simulink model "ShortPulse"  (R2018a)
settings: Solver=ode8  StartTime=0.0  StopTime=Ttot  FixedStep=Ts  RelTol=1e-3
values from neighbouring files (symbols this model uses):
  Fn = 60    [Equivalency_Script.m]    (also in FreqAdaptiveFFT_Script.m; FreqAdaptive_Script.m; ShortPulse_Script.m)
  Ts = Ts_control / 60    (= 9.25925925926e-07)    [Equivalency_Script.m]    (also in FreqAdaptiveFFT_Script.m; FreqAdaptive_Script.m; ShortPulse_Script.m)
  Ts_control = 1/(300*Fn)    (= 5.55555555556e-05)    [Equivalency_Script.m]    (also in FreqAdaptiveFFT_Script.m; FreqAdaptive_Script.m; ShortPulse_Script.m)
libraries: powerlib x3, DSCdq_Library x3, powerlib_meascontrol x1
settings Model: SimulationMode=accelerator  Creator=daniemot  LastModifiedBy=daniemot
settings SolverCC: AutoInsertRateTranBlk=on
settings DataIOCC: ExternalInput=getinputstruct(WN_50mF_op_snapshot1)  InitialState=getstatestruct(WN_50mF_op_snapshot1)  SaveFinalState=on  SaveFormat=StructureWithTime  SaveOutput=off  SignalLogging=off  DSMLogging=off  SaveTime=off
settings DebuggingCC: ReadBeforeWriteMsg=DisableAll  WriteAfterWriteMsg=DisableAll  WriteAfterReadMsg=DisableAll  MultiTaskDSMMsg=none  UnconnectedInputMsg=none  UnconnectedOutputMsg=none  UnconnectedLineMsg=none
settings ModelReferenceCC: UpdateModelReferenceTargets=IfOutOfDate
settings SFSimCC: SFSimEcho=off

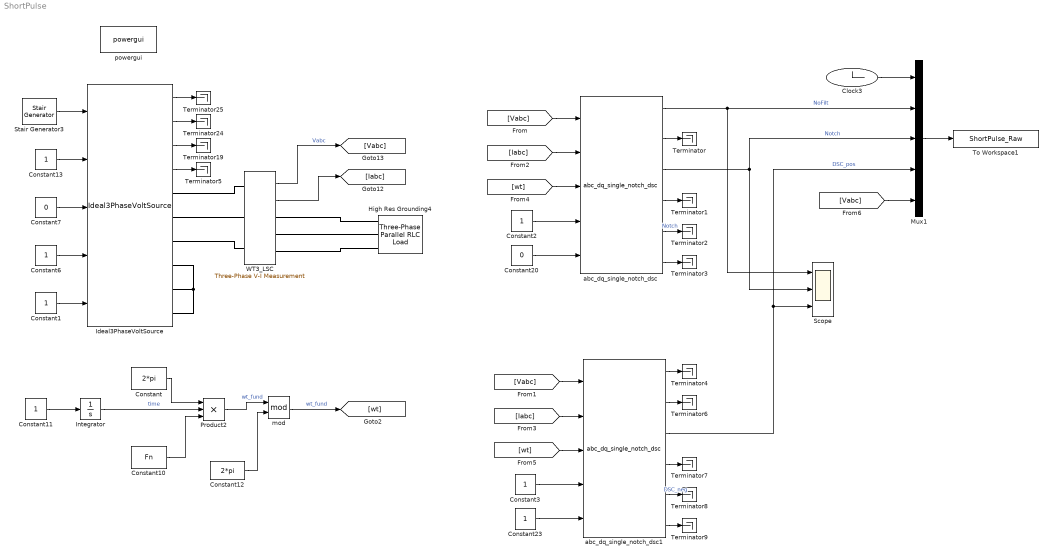
== system ShortPulse ==
  Clock3 : Clock
  Constant : Constant  Value=2*pi
  Constant{1..3,6,11,13,23} (7 alike) : Constant
  Constant10 : Constant  Value=Fn
  Constant12 : Constant  Value=2*pi
  Constant20 : Constant  Value=0
  Constant7 : Constant  Value=0
  High Res Grounding4 : powerlib/Elements/Three-Phase Parallel RLC Load  LConnTagsString=A|B|C  Configuration=Y (grounded)  NominalVoltage=(1/2^0.5)*3^0.5  Vabc=[1e3 1e3 1e3]  Vabcp=[1e3 1e3 1e3]  NominalFrequency=Fn  UnbalancedPower=off  ActivePower=3/2  InductivePower=0  CapacitivePower=0  Pabc=[10e3 9e3 11e3]  QLabc=[100 90 110]  QCabc=[100 90 110]  Pabcp=[10e3 9e3 11e3]  QLabcp=[100 90 110]  QCabcp=[100 90 110]  Measurements=None  LoadType=constant Z
  Ideal3PhaseVoltSource : DSCdq_Library/Ideal3PhaseVoltSource  BaseAmp=1  fn=Fn
  Integrator : Integrator
  Mux1 : Mux  Inputs=5
  Product2 : Product  Inputs=3
  Scope : Scope  NumInputPorts=3
  Stair Generator3 : powerlib_meascontrol/Pulse & Signal Generators/Stair Generator  t=Bench.StepTimes  e=Bench.StepValues  Ts=0
      settings: SourceProductName=Simscape Power Systems
  Terminator{,1..9,19,24..25} (13 alike) : Terminator
  To Workspace1 : ToWorkspace  VariableName=ShortPulse_Raw  SampleTime=Ts_control
      settings: Save2DSignal=2-D array (concatenate along first dimension)
  WT3_LSC : powerlib/Measurements/Three-Phase V-I Measurement  VoltageMeasurement=phase-to-ground  SetLabelV=off  LabelV=vgrid  Vpu=off  VpuLL=off  CurrentMeasurement=yes  SetLabelI=off  LabelI=igrid  Ipu=off  Pbase=sn  Vbase=uab  OutputType=Complex  PhasorSimulation=off  PSBequivalent=0
  abc_dq_single_notch_dsc : DSCdq_Library/abc_dq_single_notch_dsc  Ts=Ts_control  fn=Fn  fmin=0.8*Fn  zeta=zeta
  abc_dq_single_notch_dsc1 : DSCdq_Library/abc_dq_single_notch_dsc  Ts=Ts_control  fn=Fn  fmin=0.8*Fn  zeta=zeta
  mod : Math  Operator=mod  SaturateOnIntegerOverflow=on
  powergui : powerlib/powergui  Priority=1  SimulationMode=Discrete  SampleTime=Ts  frequency=60  Iterations=50  frequencyindice=0  Pbase=100e6  ErrMax=1e-4  UnitsV=kV  UnitsW=MW  buscounter=0  FunctionMessages=off  echomessages=off  EnableUseOfTLC=off  CurrentSourceSwitches=off  DisableSnubberDevices=off  DisableRonSwitches=off  DisableVfSwitches=off  DisplayEquations=off  SolverType=Tustin/Backward Euler (TBE)  Interpol=off  ExternalGateDelay=off  methode=off  Ts=100  x0status=blocks  SPID=off  SwTol=0  HookPort=off  RestoreLinks=warning  ResistiveCurrentMeasurement=off  Frange=[60:1:1600]  Ylog=on  Xlog=on  ShowGrid=on  save=off  variable=ZData  structure=0  ZoomFFT=off  StartTime=0.0  cycles=1  DisplayStyle=1  fundamental=60  FreqAxis=off  MaxFrequency=1000  frequencyindicesteady=1  RmsSteady=1  display=off
  wires:
  Constant6/1 -> Ideal3PhaseVoltSource/4
  Constant7/1 -> Ideal3PhaseVoltSource/3
  Constant13/1 -> Ideal3PhaseVoltSource/2
  Ideal3PhaseVoltSource/3 -> Terminator19/1
  Ideal3PhaseVoltSource/2 -> Terminator24/1
  Ideal3PhaseVoltSource/1 -> Terminator25/1
  WT3_LSC/1 -> [Vabc]  "Vabc"
  Ideal3PhaseVoltSource/4 -> Terminator5/1
  Clock3/1 -> Mux1/1
  Stair Generator3/1 -> Ideal3PhaseVoltSource/1
  abc_dq_single_notch_dsc/1 -> Mux1/2, Scope/1  "NoFilt"
  Constant20/1 -> abc_dq_single_notch_dsc/5
  Constant1/1 -> Ideal3PhaseVoltSource/5
  Constant23/1 -> abc_dq_single_notch_dsc1/5
  [Vabc] -> abc_dq_single_notch_dsc/1
  [Vabc] -> abc_dq_single_notch_dsc1/1
  [Iabc] -> abc_dq_single_notch_dsc/2
  [Iabc] -> abc_dq_single_notch_dsc1/2
  [wt] -> abc_dq_single_notch_dsc/3
  [wt] -> abc_dq_single_notch_dsc1/3
  Constant2/1 -> abc_dq_single_notch_dsc/4
  Constant3/1 -> abc_dq_single_notch_dsc1/4
  abc_dq_single_notch_dsc/3 -> Scope/2, Mux1/3  "Notch"
  abc_dq_single_notch_dsc1/3 -> Scope/3, Mux1/4  "DSC_pos"
  abc_dq_single_notch_dsc/2 -> Terminator/1
  abc_dq_single_notch_dsc/4 -> Terminator1/1
  abc_dq_single_notch_dsc/6 -> Terminator3/1
  abc_dq_single_notch_dsc1/1 -> Terminator4/1
  abc_dq_single_notch_dsc1/2 -> Terminator6/1
  abc_dq_single_notch_dsc1/4 -> Terminator7/1
  abc_dq_single_notch_dsc1/6 -> Terminator9/1
  WT3_LSC/2 -> [Iabc]
  mod/1 -> [wt]  "wt_fund"
  Constant/1 -> Product2/1
  Constant11/1 -> Integrator/1
  Integrator/1 -> Product2/2  "time"
  Constant10/1 -> Product2/3
  Constant12/1 -> mod/2
  Product2/1 -> mod/1  "wt_fund"
  abc_dq_single_notch_dsc/5 -> Terminator2/1  "Notch"
  abc_dq_single_notch_dsc1/5 -> Terminator8/1  "DSC_neg"
  Mux1/1 -> To Workspace1/1
  [Vabc] -> Mux1/5
  connections:
  Ideal3PhaseVoltSource/RConn5 -- Ideal3PhaseVoltSource/RConn6 -- Ideal3PhaseVoltSource/RConn4
  Ideal3PhaseVoltSource/RConn1 -- WT3_LSC/LConn1
  Ideal3PhaseVoltSource/RConn3 -- WT3_LSC/LConn3
  Ideal3PhaseVoltSource/RConn2 -- WT3_LSC/LConn2
  High Res Grounding4/LConn1 -- WT3_LSC/RConn1
  High Res Grounding4/LConn2 -- WT3_LSC/RConn2
  High Res Grounding4/LConn3 -- WT3_LSC/RConn3
